simulink model "Grua_MC_R2_FFLimitado_06102026"  (R2025b)
settings: Solver=ode23t  StartTime=0.0  StopTime=628  MaxStep=T_s  RelTol=1e-4
InitFcn:
  | addpath(fileparts(get_param('Grua_MC_R2_FFLimitado_06102026','FileName')),'-begin');
  | run(fullfile(fileparts(get_param('Grua_MC_R2_FFLimitado_06102026','FileName')),'definir_buses_variadores.m'));
  | run(fullfile(fileparts(get_param('Grua_MC_R2_FFLimitado_06102026','FileName')),'parametros_ganancias_cascada_29072026.m'));
  | run(fullfile(fileparts(get_param('Grua_MC_R2_FFLimitado_06102026','FileName')),'configurar_modelo_final_hmi.m'));
  | run(fullfile(fileparts(get_param('Grua_MC_R2_FFLimitado_06102026','FileName')),'configurar_parametros_variadores.m'));
  | 
  | 
  | 
  | 
  | 
  | 
  | 
  | Pvis.Ts_viz=.04;Pvis.enable=true;Pvis.keepFigureOnTerminate=true;Pvis.hmi.captureFolder='D:\AyCD\Chat\Proyecto_grua\Prueba_Completa_MC_20261007\corrida_09';Pvis.hmi.fastDiagnostic=false;Pvis.hmi.testDriver=@operador_dos_traslados_v4;Pvis.hmi.renderPeriod=.20;
StopFcn:
  | guardar_prueba_completa;
undefined symbols (not defined in the file): b_cx, b_cy, b_hb, b_hEb, b_heq, b_t, b_tb, b_teq, b_tw, b_wu, g, H_c, HMI, i_h, i_t, J_heq, J_teq, K_cy, K_tw, k_wu, L_h0, l_hi, M_c_profile, M_s, M_t, MC_FF, nLevels0, omega_hmRATED, r_hd, r_td, slotBlock, T_hbMax, T_hEbMax, T_hmMax, T_s, T_s1, T_tbMax, T_tmMax, tau_hm, tau_tm, traj_duration, traj_x_start, traj_x_target, v_hmaxLoaded, v_hmaxUnloaded, x_tmax, x_tmin, Y_c0, Y_t0, Zbase
libraries: simulink x1, aerolibanimutils x1
(part 5 of 5)

== stateflow chart Grua_MC_R2_FFLimitado_06102026/PICK // PLACE ==
  state INICIO
    entry:
    evento_cambio = false;
    tipo_evento = 0;
    slot_evento = -1;
    slot_mem = -1;
    carga_tomada = TLK;
  state VACIO1
    during:
    evento_cambio = false;
    tipo_evento = 0;
    slot_evento = -1;
    carga_tomada = 0;
  state PRE_PLACE
    during:
    evento_cambio = false;
    tipo_evento = 0;
    slot_evento = -1;
    carga_tomada = 1;
  state CARGADO1
    during:
    evento_cambio = false;
    tipo_evento = 0;
    slot_evento = -1;
    carga_tomada = 1;
  state PRE_PICK
    during:
    evento_cambio = false;
    tipo_evento = 0;
    slot_evento = -1;
    carga_tomada = 0;
  (default) -> ? [commented out]
  (default) -> ? [commented out] : [slot_ok && TLK == 1 && tension && ~contacto && v_yl > -0.05]{slot_evento = k_slot;}
  (default) -> ? [commented out] : [slot_ok && TLK == 0 && ~tension && contacto && abs(v_yl) < 0.05]{slot_evento = k_slot;}
  (default) -> ? [commented out] : [true]
  (default) -> INICIO
  INICIO -> VACIO1 [order 1] : [TLK==0]
  INICIO -> CARGADO1 [order 2] : [TLK ==1]
  PRE_PLACE -> VACIO1 [order 2] : [slot_ok && TLK == 0 && contacto]{evento_cambio = true; tipo_evento = 2; slot_evento = slot_mem;}
  CARGADO1 -> PRE_PLACE : [slot_ok && TLK == 1 && contacto && abs(v_yl) < 0.05]{slot_mem = k_slot;}
  PRE_PICK -> VACIO1 [order 1] : [~slot_ok || (~contacto && TLK == 0)]{slot_mem = -1;}
  PRE_PLACE -> CARGADO1 [order 1] : [TLK == 1 && tension && ~contacto && v_yl > 0.05]{slot_mem = -1;}
  VACIO1 -> PRE_PICK : [slot_ok && contacto && TLK == 0]{slot_mem = k_slot;}
  PRE_PICK -> CARGADO1 [order 2] : [slot_ok && TLK == 1 && tension && ~contacto && v_yl > 0.05]{evento_cambio = true; tipo_evento = 1; slot_evento = slot_mem;}
  data: TLK input; k_slot input; slot_ok input; v_yl input; evento_cambio output; tipo_evento output; slot_evento output int32; contacto input; tension input; slot_mem local int32; carga_tomada output

== matlab function Grua_MC_R2_FFLimitado_06102026/Histeresis_F_hw ==
  data: F_hw input; tension output
function tension = tension_hist_Fhw(F_hw)
% Histeresis física para detectar "cable cargado" a partir de F_hw [N].
% Basada en fracciones del peso mínimo (spreader + contenedor vacío).

% --- Parámetros físicos ---
g = 9.81;
M_s    = 15000;   % kg
M_cmin = 2000;    % kg

Wmin = (M_s + M_cmin) * g;     % N  ~ 167 kN

% --- Umbrales con histéresis ---
Fhw_on  = 0.21 * Wmin;         % ~ 35 kN (cable claramente cargado)
Fhw_off = 0.09 * Wmin;         % ~ 15 kN (cable claramente descargado)

% --- Estado persistente ---
persistent t
if isempty(t)
    t = false;
end

% --- Lógica de histéresis ---
if ~t
    if F_hw > Fhw_on
        t = true;
    end
else
    if F_hw < Fhw_off
        t = false;
    end
end

tension = t;
end

== matlab function Grua_MC_R2_FFLimitado_06102026/Histeresis_contacto ==
  data: F_cy input; contacto output
function contacto = contacto_hist_Fcy(F_cy)
% Histeresis física para detectar contacto a partir de F_cy [N].
% Basada en fracciones del peso mínimo (spreader + contenedor vacío).

% --- Parámetros físicos ---
g = 9.81;
M_s    = 15000;   % kg
M_cmin = 2000;    % kg

Wmin = (M_s + M_cmin) * g;     % N  ~ 167 kN

% --- Umbrales con histéresis ---
Fcy_on  = 0.03  * Wmin;        % ~ 5 kN (entra a contacto)
Fcy_off = 0.012 * Wmin;        % ~ 2 kN (sale de contacto)

% --- Estado persistente ---
persistent c
if isempty(c)
    c = false;
end

% --- Lógica de histéresis ---
if ~c
    if F_cy > Fcy_on
        c = true;
    end
else
    if F_cy < Fcy_off
        c = false;
    end
end

contacto = c;
end

== matlab function Grua_MC_R2_FFLimitado_06102026/slot_x_l ==
  data: x_l input; k_slot output; slot_ok output; slotBlock input
function [k_slot, slot_ok] = xl_a_slot(x_l, slotBlock)
%#codegen

x0 = -30.0;
slotWidth = 2.44;
Nslots = int32(length(slotBlock));

k = int32(1) + int32(floor((x_l - x0) / slotWidth));

if (k < 1) || (k > Nslots)
    k_slot = int32(-1);
    slot_ok = false;
else
    k_slot = k;
    slot_ok = ~slotBlock(k_slot);
end

end

== matlab function Grua_MC_R2_FFLimitado_06102026/Actualizar_Yc/update_perfil_std ==
  data: nLevels input; nLevels_new output; tipo_evento input; slot_evento input; Y_c output; Zbase input; slotBlock input; h_std input
function [nLevels_new, Y_c] = update_profile_std(nLevels, tipo_evento, slot_evento, Zbase, slotBlock, h_std)
% UPDATE_PROFILE_STD
% Actualiza el perfil discreto de obstáculos.
% Convención:
%   Y_c(k)       = altura absoluta física del tope del obstáculo.
%   nLevels(k)  = cantidad de containers en el slot k.
%   Zbase(k)    = base física absoluta del slot k.
%   slotBlock(k)= true si el slot no es operable.
%
% tipo_evento:
%   0 = NONE
%   1 = PICK
%   2 = PLACE

Nslots = int32(length(nLevels));

nLevels_new = nLevels;

slot = int32(slot_evento);

slot_ok = (slot >= 1) && (slot <= Nslots) && (~slotBlock(slot));

if slot_ok
    if tipo_evento == 1
        nLevels_new(slot) = max(nLevels_new(slot) - 1, 0);

    elseif tipo_evento == 2
        nLevels_new(slot) = nLevels_new(slot) + 1;
    end

end

Y_c = Zbase + double(nLevels_new) * h_std;

% En slots bloqueados no se codifica bloqueo dentro de Y_c.
% Se deja una altura neutral coherente con Zbase.
Y_c(slotBlock) = Zbase(slotBlock);

end

== stateflow chart Grua_MC_R2_FFLimitado_06102026/Trayectoria ==
  settings: updateMethod=DISCRETE  sampleTime=T_s  description=Generador parametrico de septimo orden. Mantiene continuas x, v, a y jerk y conserva la interfaz original.
  state Perfil_suave
    during:
    tau = elapsed/traj_duration;
    if tau > 1
    tau = 1;
    end
    delta_x = traj_x_target-traj_x_start;
    sigma = 35*tau^4-84*tau^5+70*tau^6-20*tau^7;
    dsigma = 140*tau^3-420*tau^4+420*tau^5-140*tau^6;
    d2sigma = 420*tau^2-1680*tau^3+2100*tau^4-840*tau^5;
    d3sigma = 840*tau-5040*tau^2+8400*tau^3-4200*tau^4;
    x_act = traj_x_start+delta_x*sigma;
    v_act = delta_x*dsigma/traj_duration;
    a_act = delta_x*d2sigma/(traj_duration^2);
    j_act = delta_x*d3sigma/(traj_duration^3);
    elapsed = elapsed+T_s;
  state Objetivo
    entry:
    x_act = traj_x_target;
    v_act = 0;
    a_act = 0;
    j_act = 0;
  state Esperando
    entry:
    elapsed = 0;
    x_act = traj_x_start;
    v_act = 0;
    a_act = 0;
    j_act = 0;
  (default) -> Esperando
  Perfil_suave -> Objetivo : [elapsed >= traj_duration]
  Esperando -> Perfil_suave : [iniciar == 1]
  data: j_k function_output; v_max function_input; a_max function_input; j_max function_input; j_min function_input; v_k function_input; a_k function_input; d_k function_output; fa_min function_input; a_min function_input; j_max function_input; j_min function_input; a_k function_input; a_1 function_input; v_k function_input; v_1 function_input; T_j2a function_output; T_j2b function_output; T_d function_output; j_k function_output; j_min function_input; j_max function_input; k function_input; k_d function_input; T_s function_input; T_d function_input; T_j2a function_input; T_j2b function_input; iniciar input double =0; v_act output double =0; x_act output double =0; a_act output double =0; j_act output double =0; traj_x_start parameter double; traj_x_target parameter double; traj_duration parameter double; T_s parameter double; elapsed local double =0; tau local double =0; delta_x local double =0; sigma local double =0; dsigma local double =0; d2sigma local double =0; d3sigma local double =0
  function j_k=calculo_jerk(v_max, a_max, j_max, j_min, v_k, a_k):
    | function j_k=calculo_jerk(v_max, a_max, j_max, j_min, v_k, a_k)
    | 
    | if ((v_k-(a_k^2)/(2*j_min))<v_max)&&(a_k<a_max)
    |     j_k = j_max;
    | elseif ((v_k-(a_k^2)/(2*j_min))<v_max)&&(a_k>=a_max)
    |     j_k = 0;
    | elseif ((v_k-(a_k^2)/(2*j_min))>=v_max)&&(a_k>0)
    |     j_k = j_min;
    | elseif ((v_k-(a_k^2)/(2*j_min))>=v_max)&&(a_k<=0)
    |     j_k = 0;
    | else
    |     j_k = 0;
    | end
  function [d_k, T_j2a, T_j2b, T_d]=calculo_dist_frenado(fa_min, a_min, j_max, j_min, a_k, a_1, v_k, v_1):
    | function [d_k, T_j2a, T_j2b, T_d]=calculo_dist_frenado(fa_min, a_min, j_max, j_min, a_k, a_1, v_k, v_1)
    | 
    | if fa_min==1
    |     T_j2a = (a_min-a_k)/j_min;
    |     T_j2b = (a_1-a_min)/j_max;
    |     T_d = (v_1-v_k)/a_min + T_j2a*(a_min-a_k)/(2*a_min) + T_j2b*(a_min-a_1)/(2*a_min);
    | else
    |     T_j2a = -a_k/j_min + sqrt((j_max-j_min)*(a_k^2*j_max-j_min*(a_1^2+2*j_max*(v_k-v_1))))/(j_min*(j_min-j_max));
    |     T_j2b = a_1/j_max + sqrt((j_max-j_min)*(a_k^2*j_max-j_min*(a_1^2+2*j_max*(v_k-v_1))))/(j_max*(j_max-j_min));
    |     T_d = T_j2a + T_j2b;
    | end
    | 
    | d_k = (a_k*T_d^2)/2 + (j_min*T_j2a*((3*T_d^2)-(3*T_d*T_j2a)+(T_j2a^2))+j_max*T_j2b^3)/6 + T_d*v_k;
  function j_k=calculo_jerk_des(j_min, j_max, k, k_d, T_s, T_d, T_j2a, T_j2b):
    | function j_k=calculo_jerk_des(j_min, j_max, k, k_d, T_s, T_d, T_j2a, T_j2b)
    | if ((k-k_d)>=0)&&((k-k_d)<(T_j2a/T_s))
    |     j_k = j_min;
    | elseif ((k-k_d)>=(T_j2a/T_s))&&((k-k_d)<((T_d-T_j2b)/T_s))
    |     j_k = 0;
    | elseif ((k-k_d)>=((T_d-T_j2b)/T_s))&&((k-k_d)<=(T_d/T_s))
    |     j_k = j_max;
    | else
    |     j_k = 0;
    | end
